simulink model "leerUARTSimulink"  (R2018a)
settings: Solver=VariableStepAuto  StartTime=0.0  StopTime=inf  RelTol=1e-3
libraries: instrumentlib x1
settings Model: Creator=LeoXtr3m  LastModifiedBy=LeoXtr3m

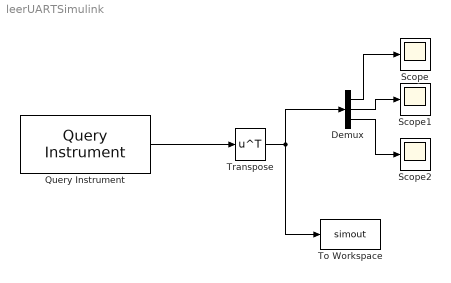
== system leerUARTSimulink ==
  Demux : Demux  Outputs=3
  Query Instrument : instrumentlib/Query Instrument  sampleTime=inf  isWorkspaceObject=off  timeout=10  inputBufferSize=512  protocol=Serial  serialPort=COM4  baudRate=9600  gpibVendor=Keysight Technologies  boardIndex=0  primaryAddress=1  secondaryAddress=0  visaVendor=Keysight  visaSerialPort=0  chassisIndex=0  logicalAddress=0  tcpRemoteHost='127.0.0.1'  tcpRemotePort=4500  udpRemoteHost='127.0.0.1'  udpRemotePort=9090  visaTCPBoardIndex=0  visaTCPRemoteHost='127.0.0.1'  usbBoardIndex=0  usbManufID=0  usbModelCode=0  usbSerialNumber=0  initAction=None  initCommand='DATA:SOURCE CH1'  initFunction=get  queryCommand='curve?'  responseFormat=ASCII  asciiFormatting='%d,%d,%d'  precision=8-bit integer  byteOrder=Little endian  valuesToRead=1  removeBytes=off  afterOutputAction=Repeat query for new data  enableFrames=on  frameSize=3
      settings: SourceProductName=Instrument Control Toolbox  SourceProductBaseCode=IC
  Scope : Scope
  Scope1 : Scope
  Scope2 : Scope
  To Workspace : ToWorkspace  VariableName=simout  SaveFormat=Timeseries  SampleTime=-1
  Transpose : Math  Operator=transpose  SaturateOnIntegerOverflow=on
  wires:
  Query Instrument/1 -> Transpose/1
  Transpose/1 -> Demux/1, To Workspace/1
  Demux/2 -> Scope1/1
  Demux/1 -> Scope/1
  Demux/3 -> Scope2/1
